simulink model "guidance_sub"  (R2017a)
settings: Solver=ode4  StartTime=0.0  StopTime=600  FixedStep=gnc_sub.guidance.dt  RelTol=1e-3
settings Model: Creator=simone  LastModifiedBy=gcstation
settings DataIOCC: SaveOutput=off  SaveTime=off
settings OptimizationCC: DefaultParameterBehavior=Inlined  PassReuseOutputArgsAs=Individual arguments
settings DebuggingCC: ParameterTunabilityLossMsg=error
settings HardwareCC: ProdBitPerLong=64  ProdHWDeviceType=Intel->x86-64 (Linux 64)
settings SFSimCC: MATLABDynamicMemAlloc=off
settings RTWCC: SystemTargetFile=ert.tlc  TemplateMakefile=ert_default_tmf  Description=Embedded Coder  GenerateReport=on  IncludeHyperlinkInReport=on  LaunchReport=on  TargetLang=C++  GenerateTraceInfo=on  GenerateTraceReport=on  GenerateTraceReportSl=on  GenerateTraceReportSf=on  GenerateTraceReportEml=on
settings CodeAppCC: ForceParamTrailComments=on  IgnoreCustomStorageClasses=off  OperatorAnnotations=on  SimulinkDataObjDesc=on  SFDataObjDesc=on  MATLABFcnDesc=on  InsertBlockDesc=on  MATLABSourceComments=on
settings ERTTargetCC: TargetLangStandard=C++03 (ISO)  GenerateSampleERTMain=on  MultiInstanceERTCode=on  CodeInterfacePackaging=C++ class  InlinedParameterPlacement=NonHierarchical  RootIOFormat=Structure reference  ERTCustomFileTemplate=example_file_process.tlc

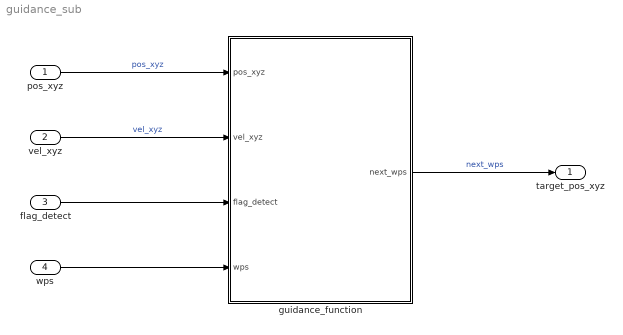
== system guidance_sub ==
  pos_xyz : Inport  OutDataTypeStr=double  PortDimensions=[3 1]  SampleTime=[0.050000000000000003,0]
  vel_xyz : Inport  Port=2  OutDataTypeStr=double  PortDimensions=[3 1]  SampleTime=[0.050000000000000003,0]
  flag_detect : Inport  Port=3  OutDataTypeStr=boolean  PortDimensions=[1 1]  SampleTime=[0.050000000000000003,0]
  wps : Inport  Port=4  OutDataTypeStr=double  PortDimensions=[3,2]
  guidance_function : MATLAB Function  TreatAsAtomicUnit=on
  target_pos_xyz : Outport  OutDataTypeStr=double  PortDimensions=[3 1]  SampleTime=[0.050000000000000003,0]
  wires:
  flag_detect/1 -> guidance_function/3(flag_detect)
  vel_xyz/1 -> guidance_function/2(vel_xyz)  "vel_xyz"
  pos_xyz/1 -> guidance_function/1(pos_xyz)  "pos_xyz"
  guidance_function/1(next_wps) -> target_pos_xyz/1  "next_wps"
  wps/1 -> guidance_function/4(wps)

== matlab function guidance_sub/guidance_function ==
  data: pos_xyz input; next_wps output size=[3,1]; vel_xyz input; flag_detect input; wps input
function next_wps = guidance_wrp(pos_xyz,vel_xyz,flag_detect,wps)
persistent j found_target target_pos

if isempty(target_pos)
    j = 1;
    target_pos = [0 0 0]';
    found_target = 0;
end

next_wps = zeros(3,1);
if ~found_target
    next_wps = wps(1:3,j);
    
    % go between wps
    if norm(pos_xyz-next_wps) < 1
        j = j+1;
        if j > 2
            j=1;
        end
        
    end
    
    % stop there
    if flag_detect 
        found_target = 1;
        target_pos = pos_xyz;
        next_wps = target_pos;
    end
else
    next_wps = target_pos;
end

    








end
